simulink model "PMSM_HFI_PulseCos_Continuouse"  (R2022b)
settings: Solver=ode45  StartTime=0.0  StopTime=3  RelTol=1e-3  EnableMultiTasking=on
libraries: dsparch4 x6, spsVoltageMeasurementLib x3, spsUniversalBridgeLib x2, spsGroundLib x1, spsPermanentMagnetSynchronousMachineLib x1, simulink x1, spsThreePhaseVIMeasurementLib x1, spsDCVoltageSourceLib x1, spspowerguiLib x1
settings Model: Creator=lovejing  LastModifiedBy=yll
settings SolverCC: ZeroCrossAlgorithm=Adaptive  AlgebraicLoopSolver=TrustRegion
settings DataIOCC: LimitDataPoints=on  SaveFormat=Array  SignalLoggingSaveFormat=ModelDataLogs  ReturnWorkspaceOutputs=off
settings OptimizationCC: ExpressionDepthLimit=2147483647  LifeSpan=inf
settings DebuggingCC: UnderspecifiedInitializationDetection=Classic  MergeDetectMultiDrivingBlocksExec=none  SolverPrmCheckMsg=warning  FcnCallInpInsideContextMsg=warning  UnconnectedInputMsg=warning  UnconnectedOutputMsg=warning  UnconnectedLineMsg=warning  StateNameClashWarn=warning  SFUnexpectedBacktrackingDiag=warning  SFNoUnconditionalDefaultTransitionDiag=warning  SFExecutionAtInitializationDiag=none  SFMachineParentedDataDiag=warning  ArithmeticOperatorsInVariantConditions=warning
settings HardwareCC: ProdBitPerPointer=32  ProdBitPerSizeT=32  ProdBitPerPtrDiffT=32  ProdLargestAtomicFloat=None  ProdIntDivRoundTo=Undefined  ProdEndianess=Unspecified  ProdWordSize=32  ProdHWDeviceType=32-bit Generic
settings ModelReferenceCC: PropagateSignalLabelsOutOfModel=off
settings SFSimCC: SimUseLocalCustomCode=off  CustomCodeUndefinedFunction=UseInterfaceOnly
settings RTWCC: RTWUseLocalCustomCode=off
settings CodeAppCC: StateflowObjectComments=on
settings GRTTargetCC: TargetLangStandard=C89/C90 (ANSI)  CombineOutputUpdateFcns=off  GRTInterface=on
settings ConfigComp: CovMetricSettings=dw  CovSaveCumulativeToWorkspaceVar=on  CovSaveSingleToWorkspaceVar=on  CovExternalEMLEnable=off  CovSFcnEnable=off
settings SimscapeCC: SimscapeNormalizeSystem=off

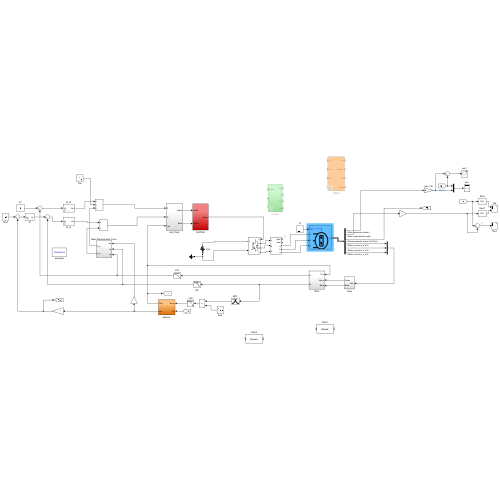
[thumbnail: Simulink's stored preview of the top-level diagram]
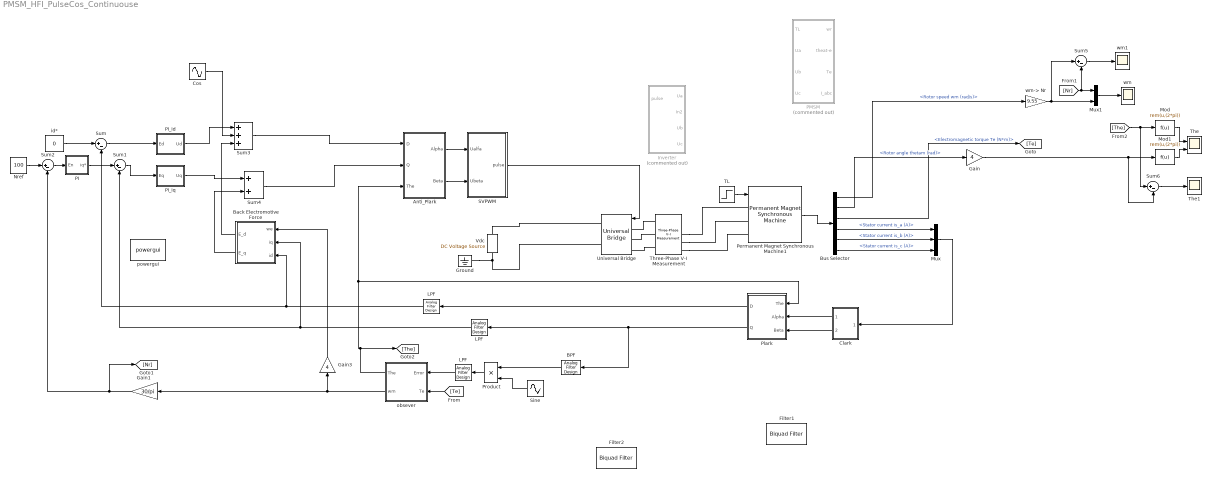
== system PMSM_HFI_PulseCos_Continuouse ==
  " LPF" : dsparch4/Analog Filter Design  method=Butterworth  filttype=Lowpass  N=1  Wlo=942  Whi=80  Rp=2  Rs=40
  Anti_Plark : Subsystem
  BPF : dsparch4/Analog Filter Design  method=Butterworth  filttype=Bandpass  N=2  Wlo=6200  Whi=6360  Rp=2  Rs=40
  Back Electromotive Force : Subsystem
  Bus Selector : BusSelector  OutputSignals=Rotor speed wm (rad/s),Rotor angle thetam (rad),Electromagnetic torque Te (N*m),Stator current is_a (A),Stator current is_b (A),Stator current is_c (A)
  Clark : Subsystem
  Cos : Sin  Amplitude=20  Frequency=6280  Phase=pi/2  SampleTime=0
  Filter1 : dsparch4/Biquad Filter  Tag=BlockMethodSubSystem  FilterSource=Dialog parameters  CoeffSource=Specify via dialog  FilterObject=BQF  IIRFiltStruct=Direct form II  BiQuadCoeffs=[1 0 -1 1 -1.99827576792918582 0.999875701454450927;1 0 -1 1 -1.99836499980206295 0.999879080975449419;1 0 -1 1 -1.99803610170332835 0.999633631467209849;1 0 -1 1 -1.99812710154029682 0.999643098504342187;1 0 -1 1 -1.99781763221036179 0.99941068343367212;1 0 -1 1 -1.99790443799382444 0.999424361176048381;1 0 -1 1 -1.99763159357438957 0.999218332257679753;1 0 -1 1 -1.99770783357569925 0.999233511136148667;1 0 -1 1 -1.99748738637941559 0.999066314462234151;1 0 -1 1 -1.99754699818338244 0.999079988713626688;1 0 -1 1 -1.9973920922120505 0.998962122228290506;1 0 -1 1 -1.99743006957830049 0.998971584387099765;1 0 -1 1 -1.99735014806338107 0.998910653324007525;1 0 -1 1 -1.99736319098991588 0.99891403010315738]  ScaleValues=[0.000547534400617177147;0.000547534400617177147;0.000547468966985179494;0.000547468966985179494;0.000547408518068997194;0.000547408518068997194;0.000547356078689129684;0.000547356078689129684;0.000547314270478672362;0.000547314270478672362;0.000547285181986175264;0.000547285181986175264;0.000547270265506675873;0.000547270265506675873;1]  IC=0  ICnum=0  ICden=0  a0Flag=Warning  optimizeScaleValues=on  ScaleValueMode=Specify via input port (g)  InputProcessing=Columns as channels (frame based)  roundingMode=Floor  overflowMode=off  scaleValueFracLength=14  denProdOutputFracLength=30  denAccumFracLength=30  secondMemoryFracLength=15
  Filter2 : dsparch4/Biquad Filter  Tag=BlockMethodSubSystem  FilterSource=Dialog parameters  CoeffSource=Specify via dialog  FilterObject=BQF  IIRFiltStruct=Direct form II  BiQuadCoeffs=[1 0 -1 1 -1.99827576792918582 0.999875701454450927;1 0 -1 1 -1.99836499980206295 0.999879080975449419;1 0 -1 1 -1.99803610170332835 0.999633631467209849;1 0 -1 1 -1.99812710154029682 0.999643098504342187;1 0 -1 1 -1.99781763221036179 0.99941068343367212;1 0 -1 1 -1.99790443799382444 0.999424361176048381;1 0 -1 1 -1.99763159357438957 0.999218332257679753;1 0 -1 1 -1.99770783357569925 0.999233511136148667;1 0 -1 1 -1.99748738637941559 0.999066314462234151;1 0 -1 1 -1.99754699818338244 0.999079988713626688;1 0 -1 1 -1.9973920922120505 0.998962122228290506;1 0 -1 1 -1.99743006957830049 0.998971584387099765;1 0 -1 1 -1.99735014806338107 0.998910653324007525;1 0 -1 1 -1.99736319098991588 0.99891403010315738]  ScaleValues=[0.000547534400617177147;0.000547534400617177147;0.000547468966985179494;0.000547468966985179494;0.000547408518068997194;0.000547408518068997194;0.000547356078689129684;0.000547356078689129684;0.000547314270478672362;0.000547314270478672362;0.000547285181986175264;0.000547285181986175264;0.000547270265506675873;0.000547270265506675873;1]  IC=0  ICnum=0  ICden=0  a0Flag=Warning  optimizeScaleValues=on  ScaleValueMode=Specify via input port (g)  InputProcessing=Columns as channels (frame based)  roundingMode=Floor  overflowMode=off  scaleValueFracLength=14  denProdOutputFracLength=30  denAccumFracLength=30  secondMemoryFracLength=15
  Gain : Gain  Gain=4
  Gain1 : Gain  Gain=30/pi
  Gain3 : Gain  Gain=4
  Ground : spsGroundLib/Ground  LConnTagsString=a
  Inverter : Subsystem  Commented=on
      settings: PortSchema="{\"entries\":[{\"content\":{\"sides\":[{\"content\":{\"connectorIds\":[\"In1\",\"LConn1\",\"LConn2\"]},\"type\":\"ConnectorPlacement.EquallySpacedRectSide\",\"uuid\":\"4e818927-345e-4f01-8e72-8098c662edc2\"},{\"content\":{\"connectorIds\":[\"Out1\",\"In2\",\"Out2\",\"Out3\"],\"side\":\"RIGHT\"},\"type\":\"ConnectorPlacement.EquallySpacedRectSide\",\"uuid\":\"f77f2109-fd93-4188-b06e-da3c9e8aa1ae\"},{\"content\":{\"connectorIds\":[],\"side\":\"TOP\"},\"type\":\"ConnectorPlacement.EquallySpacedRectSide\",\"uuid\":\"a2773a45-0f31-47fa-94c1-50539ffbc16b\"}]},\"type\":\"ConnectorPlacement.EquallySpacedConnector\",\"uuid\":\"32311cb9-9857-42c7-bd27-5d83894cf80f\"}],\"packageUris\":[\"http://schema.mathworks.com/mf0/Connector/R2020b\"],\"version\":\"1.0\"}"
  LPF : dsparch4/Analog Filter Design  method=Butterworth  filttype=Lowpass  N=1  Wlo=942  Whi=80  Rp=2  Rs=40
  "LPF " : dsparch4/Analog Filter Design  method=Butterworth  filttype=Lowpass  N=1  Wlo=942  Whi=80  Rp=2  Rs=40
  Mod : Fcn  Expr=rem(u,(2*pi))
  Mod1 : Fcn  Expr=rem(u,(2*pi))
  Mux : Mux  Inputs=3
  Mux1 : Mux  Inputs=2
  Nref : Constant  Value=100
  PI : Subsystem  mask{Knp=0.4, Kni=2}
  PI_id : Subsystem  mask{Kip=40, Kii=1}
  PI_iq : Subsystem  mask{Kip=40, Kii=1}
  PMSM : Subsystem  Commented=on  mask{Ld=0.0052, R=0.33, Lq=0.0174, kf=0.646, p=2, F=0, J=0.008}
  Permanent Magnet Synchronous Machine1 : spsPermanentMagnetSynchronousMachineLib/Permanent Magnet Synchronous Machine  NbPhases=3  FluxDistribution=Sinusoidal  RotorType=Salient-pole  MechanicalLoad=Torque Tm  PresetModel=No  ShowDetailedParameters=on  MeasurementBus=off  Resistance=0.02  Inductance=8.5e-3  dqInductances=[0.002 0.004]  La=Motor_Ld_Indctances  MachineConstant=Flux linkage established by magnets (V.s)  Flux=0.08  VoltageCst=58.0416  TorqueCst=0.48  Flat=120  Mechanical=[0.003 0 4 0]  PolePairs=4  InitialConditions=[0,0,0,0]  InitialConditions5ph=[0 0 0 0 0 0]  RefAngle=Aligned with phase A axis (original Park)  IterativeDiscreteModel=Trapezoidal robust  TsBlock=-1  TsPowergui=0
  Plark : Subsystem
  Product : Product
  SVPWM : Subsystem
  "Sine " : Sin  Frequency=6280  SampleTime=0
  Sum{,1..2,5..6} (5 alike) : Sum  Inputs=|+-
  Sum3 : Sum  Inputs=+++
  Sum4 : Sum
  TL : Step  Time=0.05  After=0  SampleTime=0
  The : Scope  NumInputPorts=2
  The1 : Scope
  Three-Phase V-I Measurement : spsThreePhaseVIMeasurementLib/Three-Phase V-I Measurement  VoltageMeasurement=phase-to-ground  SetLabelV=off  LabelV=Vabc  Vpu=off  VpuLL=off  CurrentMeasurement=yes  SetLabelI=off  LabelI=Iabc  Ipu=off  Pbase=100e6  Vbase=500e3  OutputType=Complex  PhasorSimulation=off  PSBequivalent=0
  Universal Bridge : spsUniversalBridgeLib/Universal Bridge  Arms=3  SnubberResistance=1e5  SnubberCapacitance=inf  Device=IGBT / Diodes  Ron=1e-3  Lon=0  ForwardVoltages="[  0  0  ]"  ForwardVoltage=0  GTOparameters=[ 10e-6 , 20e-6 ]  IGBTparameters=[ 1e-6 , 2e-6 ]  Measurements=None  Measurements_2=None  converterType=Rectifier
  "Vdc " : spsDCVoltageSourceLib/DC Voltage Source  Amplitude=311  Measurements=None
  id* : Constant  Value=0
  obsever : Subsystem
  powergui : spspowerguiLib/powergui  Priority=1  SimulationMode=Continuous  SampleTime=1e-6  frequency=60  Iterations=50  frequencyindice=0  Pbase=100e6  ErrMax=1e-4  UnitsV=kV  UnitsW=MW  buscounter=0  FunctionMessages=off  echomessages=off  EnableUseOfTLC=off  CurrentSourceSwitches=off  DisableSnubberDevices=off  DisableRonSwitches=off  DisableVfSwitches=off  DisplayEquations=off  AutomaticDiscreteSolvers=off  SolverType=Tustin/Backward Euler (TBE)  Interpol=off  ExternalGateDelay=off  methode=off  Ts=100  x0status=blocks  SPID=off  SwTol=0  HookPort=off  NonlinearTolerance=1e-4  nMaxIteration=100  ContinueOnMaxIteration=off  RestoreLinks=warning  ResistiveCurrentMeasurement=off  Frange=[0:2:500]  Ylog=off  Xlog=on  ShowGrid=off  save=off  variable=ZData  structure=0  ZoomFFT=off  StartTime=0.0  cycles=1  DisplayStyle=1  fundamental=60  FreqAxis=off  MaxFrequency=1000  frequencyindicesteady=1  RmsSteady=1  display=off
  wm : Scope
  wm-> Nr : Gain  Gain=9.55
  wm1 : Scope
  wires:
  Gain/1 -> Sum6/2, Mod1/1
  Bus Selector/3 -> [Te]  "<Electromagnetic torque Te (N*m)>"
  Bus Selector/4 -> Mux/1  "<Stator current is_a (A)>"
  TL/1 -> Permanent Magnet Synchronous Machine1/1
  BPF/1 -> Product/1
  SVPWM/1(pulse) -> Universal Bridge/1
  " LPF"/1 -> obsever/1(Error)
  [Te] -> obsever/2(Te)
  "Sine "/1 -> Product/2
  wm-> Nr/1 -> Sum5/1, Mux1/2
  [The] -> Sum6/1, Mod/1
  [Nr] -> Sum5/2, Mux1/1
  Plark/2(Q) -> BPF/1, "LPF "/1
  Gain1/1 -> [Nr], Sum2/2
  PI/1(iq*) -> Sum1/1
  "LPF "/1 -> Back Electromotive Force/2(iq), Sum1/2
  id*/1 -> Sum/1
  Plark/1(D) -> LPF/1
  Mod/1 -> The/1
  Sum3/1 -> Anti_Plark/1(D)
  Anti_Plark/1(Alpha) -> SVPWM/1(Ualfa)
  Clark/2(Beta) -> Plark/3(Beta)
  Mux1/1 -> wm/1
  Clark/1(Alpha) -> Plark/2(Alpha)
  Sum5/1 -> wm1/1
  PI_id/1(Ud) -> Sum3/1
  LPF/1 -> Back Electromotive Force/3(id), Sum/2
  Permanent Magnet Synchronous Machine1/1 -> Bus Selector/1
  Sum1/1 -> PI_iq/1(Eq)
  Sum/1 -> PI_id/1(Ed)
  Sum2/1 -> PI/1(En)
  Nref/1 -> Sum2/1
  Anti_Plark/2(Beta) -> SVPWM/2(Ubeta)
  Bus Selector/2 -> Gain/1  "<Rotor angle thetam (rad)>"
  Bus Selector/6 -> Mux/3  "<Stator current is_c (A)>"
  Bus Selector/5 -> Mux/2  "<Stator current is_b (A)>"
  Mod1/1 -> The/2
  obsever/1(The) -> [The], Plark/1(The), Anti_Plark/3(The)
  Product/1 -> " LPF"/1
  Mux/1 -> Clark/1(ABC)
  Sum6/1 -> The1/1
  Bus Selector/1 -> wm-> Nr/1  "<Rotor speed wm (rad/s)>"
  Cos/1 -> Sum3/2
  Sum4/1 -> Anti_Plark/2(Q)
  PI_iq/1(Uq) -> Sum4/1
  Back Electromotive Force/1(E_d) -> Sum3/3
  Back Electromotive Force/2(E_q) -> Sum4/2
  obsever/2(wm) -> Gain3/1, Gain1/1
  Gain3/1 -> Back Electromotive Force/1(we)
  connections:
  "Vdc "/LConn1 -- Universal Bridge/RConn2 -- Ground/LConn1
  Universal Bridge/RConn1 -- "Vdc "/RConn1
  Three-Phase V-I Measurement/LConn2 -- Universal Bridge/LConn2
  Three-Phase V-I Measurement/RConn1 -- Permanent Magnet Synchronous Machine1/LConn1
  Three-Phase V-I Measurement/RConn2 -- Permanent Magnet Synchronous Machine1/LConn2
  Three-Phase V-I Measurement/LConn3 -- Universal Bridge/LConn3
  Three-Phase V-I Measurement/RConn3 -- Permanent Magnet Synchronous Machine1/LConn3
  Three-Phase V-I Measurement/LConn1 -- Universal Bridge/LConn1

== system PMSM_HFI_PulseCos_Continuouse/Anti_Plark ==
  D : Inport
  Q : Inport  Port=2
  The : Inport  Port=3
  Mux : Mux  Inputs=3
  alpha : Fcn  Expr=u(1)*cos(u(3))-u(2)*sin(u(3))
  beta : Fcn  Expr=u(1)*sin(u(3))+u(2)*cos(u(3))
  Alpha : Outport
  Beta : Outport  Port=2
  wires:
  alpha/1 -> Alpha/1
  Q/1 -> Mux/2
  The/1 -> Mux/3
  D/1 -> Mux/1
  Mux/1 -> beta/1, alpha/1
  beta/1 -> Beta/1

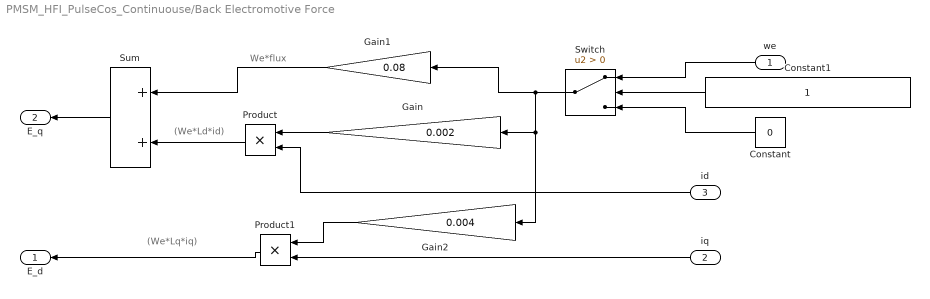
== system PMSM_HFI_PulseCos_Continuouse/Back Electromotive Force ==
  note: (We*Ld*id)
  note: We*flux
  note: (We*Lq*iq)
  we : Inport
  iq : Inport  Port=2
  id : Inport  Port=3
  Constant : Constant  Value=0
  Constant1 : Constant
  Gain : Gain  Gain=0.002
  Gain1 : Gain  Gain=0.08
  Gain2 : Gain  Gain=0.004
  Product : Product
  Product1 : Product
  Sum : Sum
  Switch : Switch  Criteria=u2 > Threshold  SaturateOnIntegerOverflow=off  InputSameDT=off
  E_d : Outport
  E_q : Outport  Port=2
  wires:
  Constant/1 -> Switch/3
  we/1 -> Switch/1
  Gain/1 -> Product/1
  Gain2/1 -> Product1/1
  iq/1 -> Product1/2
  id/1 -> Product/2
  Constant1/1 -> Switch/2
  Product/1 -> Sum/2
  Sum/1 -> E_q/1
  Gain1/1 -> Sum/1
  Product1/1 -> E_d/1
  Switch/1 -> Gain2/1, Gain/1, Gain1/1

== system PMSM_HFI_PulseCos_Continuouse/Clark ==
  ABC : Inport
  alpha : Fcn  Expr=(u(1)-0.5*(u(2)+u(3)))*2/3
  beta : Fcn  Expr=sqrt(3)/2*(u(2)-u(3))*2/3
  Alpha : Outport
  Beta : Outport  Port=2
  wires:
  alpha/1 -> Alpha/1
  ABC/1 -> beta/1, alpha/1
  beta/1 -> Beta/1

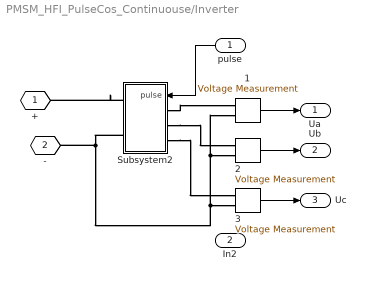
== system PMSM_HFI_PulseCos_Continuouse/Inverter ==
  pulse : Inport
  In2 : Inport  Port=2
  1 : spsVoltageMeasurementLib/Voltage Measurement  PhasorSimulation=off  OutputType=Complex  PSBequivalent=0
  2 : spsVoltageMeasurementLib/Voltage Measurement  PhasorSimulation=off  OutputType=Complex  PSBequivalent=0
  3 : spsVoltageMeasurementLib/Voltage Measurement  PhasorSimulation=off  OutputType=Complex  PSBequivalent=0
  Subsystem2 : Subsystem
  + : PMIOPort  Tag=PMCPort  Side=Left
  - : PMIOPort  Tag=PMCPort  Port=2  Side=Left
  Ua : Outport
  Ub : Outport  Port=2
  Uc : Outport  Port=3
  wires:
  3/1 -> Uc/1
  2/1 -> Ub/1
  1/1 -> Ua/1
  pulse/1 -> Subsystem2/1(pulse)
  connections:
  Subsystem2/LConn1 -- 1/LConn1
  -/RConn1 -- Subsystem2/RConn2 -- 3/LConn2 -- 2/LConn2 -- 1/LConn2
  Subsystem2/LConn2 -- 2/LConn1
  Subsystem2/LConn3 -- 3/LConn1
  Subsystem2/RConn1 -- +/RConn1

== system PMSM_HFI_PulseCos_Continuouse/PI ==
  En : Inport
  Gain : Gain  Gain=Kni
  Gain1 : Gain  Gain=Knp
  Integrator : Integrator
  Saturation : Saturate  UpperLimit=50  LowerLimit=-50
  Subtract : Sum
  iq* : Outport
  wires:
  En/1 -> Gain/1, Gain1/1
  Gain/1 -> Integrator/1
  Integrator/1 -> Subtract/1
  Gain1/1 -> Subtract/2
  Subtract/1 -> Saturation/1
  Saturation/1 -> iq*/1

== system PMSM_HFI_PulseCos_Continuouse/PI_id ==
  Ed : Inport
  Gain : Gain  Gain=Kii
  Gain1 : Gain  Gain=Kip
  Integrator : Integrator
  Saturation : Saturate  UpperLimit=10  LowerLimit=-10
  Subtract : Sum
  Ud : Outport
  wires:
  Ed/1 -> Gain/1, Gain1/1
  Gain/1 -> Integrator/1
  Integrator/1 -> Subtract/1
  Gain1/1 -> Subtract/2
  Subtract/1 -> Saturation/1
  Saturation/1 -> Ud/1

== system PMSM_HFI_PulseCos_Continuouse/PI_iq ==
  Eq : Inport
  Gain : Gain  Gain=Kii
  Gain1 : Gain  Gain=Kip
  Integrator : Integrator
  Saturation : Saturate  UpperLimit=100  LowerLimit=-100
  Subtract : Sum
  Uq : Outport
  wires:
  Eq/1 -> Gain/1, Gain1/1
  Gain/1 -> Integrator/1
  Integrator/1 -> Subtract/1
  Gain1/1 -> Subtract/2
  Subtract/1 -> Saturation/1
  Saturation/1 -> Uq/1

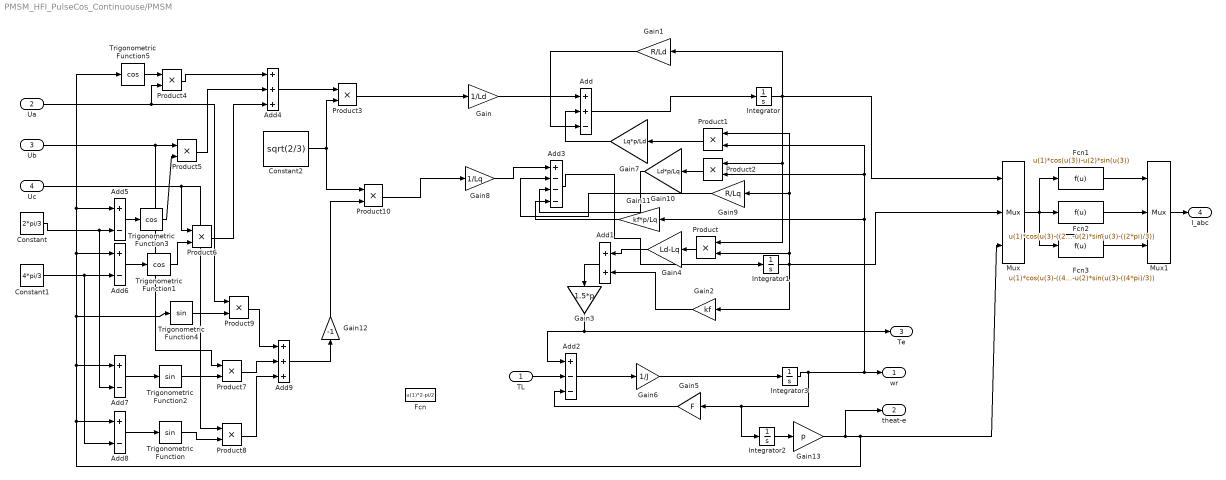
== system PMSM_HFI_PulseCos_Continuouse/PMSM ==
  TL : Inport
  Ua : Inport  Port=2
  Ub : Inport  Port=3
  Uc : Inport  Port=4
  Add : Sum  Inputs=++-
  Add1 : Sum
  Add2 : Sum  Inputs=+--
  Add3 : Sum  Inputs=+---
  Add4 : Sum  Inputs=+++
  Add{5..8} (4 alike) : Sum  Inputs=+-
  Add9 : Sum  Inputs=+++
  Constant : Constant  Value=2*pi/3
  Constant1 : Constant  Value=4*pi/3
  Constant2 : Constant  Value=sqrt(2/3)
  Fcn : Fcn  Expr=u(1)*2-pi/2
  Fcn1 : Fcn  Expr=u(1)*cos(u(3))-u(2)*sin(u(3))
  Fcn2 : Fcn  Expr=u(1)*cos(u(3)-((2*pi)/3))-u(2)*sin(u(3)-((2*pi)/3))
  Fcn3 : Fcn  Expr=u(1)*cos(u(3)-((4*pi)/3))-u(2)*sin(u(3)-((4*pi)/3))
  Gain : Gain  Gain=1/Ld
  Gain1 : Gain  Gain=R/Ld
  Gain10 : Gain  Gain=Ld*p/Lq
  Gain11 : Gain  Gain=kf*p/Lq
  Gain12 : Gain  Gain=-1
  Gain13 : Gain  Gain=p
  Gain2 : Gain  Gain=kf
  Gain3 : Gain  Gain=1.5*p
  Gain4 : Gain  Gain=Ld-Lq
  Gain5 : Gain  Gain=F
  Gain6 : Gain  Gain=1/J
  Gain7 : Gain  Gain=Lq*p/Ld
  Gain8 : Gain  Gain=1/Lq
  Gain9 : Gain  Gain=R/Lq
  Integrator{,1..3} (4 alike) : Integrator
  Mux : Mux  Inputs=3
  Mux1 : Mux  Inputs=3
  Product{,1..10} (11 alike) : Product  RndMeth=Zero
  Trigonometric Function : Trigonometry
  Trigonometric Function1 : Trigonometry  Operator=cos
  Trigonometric Function2 : Trigonometry
  Trigonometric Function3 : Trigonometry  Operator=cos
  Trigonometric Function4 : Trigonometry
  Trigonometric Function5 : Trigonometry  Operator=cos
  wr : Outport
  theat-e : Outport  Port=2
  Te : Outport  Port=3
  I_abc : Outport  Port=4
  wires:
  Add3/1 -> Integrator1/1
  Gain11/1 -> Add3/4
  Gain10/1 -> Add3/3
  Product2/1 -> Gain10/1
  Gain9/1 -> Add3/2
  Gain8/1 -> Add3/1
  Add/1 -> Integrator/1
  Gain7/1 -> Add/2
  Product1/1 -> Gain7/1
  Gain6/1 -> Integrator3/1
  Add2/1 -> Gain6/1
  Gain5/1 -> Add2/3
  TL/1 -> Add2/2
  Integrator3/1 -> wr/1, Product1/2, Product2/2, Gain11/1, Gain5/1, Integrator2/1
  Gain3/1 -> Add2/1, Te/1
  Add1/1 -> Gain3/1
  Gain2/1 -> Add1/2
  Gain4/1 -> Add1/1
  Product/1 -> Gain4/1
  Gain1/1 -> Add/3
  Integrator1/1 -> Product/2, Product1/1, Gain9/1, Gain2/1, Mux/2
  Integrator/1 -> Gain1/1, Product/1, Product2/1, Mux/1
  Gain/1 -> Add/1
  Constant2/1 -> Product3/2, Product10/1
  Add4/1 -> Product3/1
  Product3/1 -> Gain/1
  Constant/1 -> Add5/2, Add7/2
  Add5/1 -> Trigonometric Function3/1
  Constant1/1 -> Add6/2, Add8/2
  Add6/1 -> Trigonometric Function1/1
  Trigonometric Function5/1 -> Product4/1
  Ua/1 -> Product4/2, Product9/1
  Product4/1 -> Add4/1
  Ub/1 -> Product5/1, Product7/1
  Trigonometric Function3/1 -> Product5/2
  Product5/1 -> Add4/2
  Uc/1 -> Product6/1, Product8/1
  Trigonometric Function1/1 -> Product6/2
  Product6/1 -> Add4/3
  Add7/1 -> Trigonometric Function2/1
  Add8/1 -> Trigonometric Function/1
  Trigonometric Function2/1 -> Product7/2
  Trigonometric Function/1 -> Product8/2
  Trigonometric Function4/1 -> Product9/2
  Product9/1 -> Add9/1
  Product7/1 -> Add9/2
  Product8/1 -> Add9/3
  Add9/1 -> Gain12/1
  Gain12/1 -> Product10/2
  Product10/1 -> Gain8/1
  Gain13/1 -> Add8/1, Add7/1, Trigonometric Function5/1, Add5/1, Add6/1, Trigonometric Function4/1, Mux/3, theat-e/1
  Fcn3/1 -> Mux1/3
  Fcn2/1 -> Mux1/2
  Fcn1/1 -> Mux1/1
  Mux/1 -> Fcn2/1, Fcn1/1, Fcn3/1
  Mux1/1 -> I_abc/1
  Integrator2/1 -> Gain13/1

== system PMSM_HFI_PulseCos_Continuouse/Plark ==
  The : Inport
  Alpha : Inport  Port=2
  Beta : Inport  Port=3
  Mux : Mux  Inputs=3
  d : Fcn  Expr=u(1)*cos(u(3))+u(2)*sin(u(3))
  q : Fcn  Expr=-u(1)*sin(u(3))+u(2)*cos(u(3))
  D : Outport
  Q : Outport  Port=2
  wires:
  d/1 -> D/1
  Beta/1 -> Mux/2
  The/1 -> Mux/3
  Alpha/1 -> Mux/1
  Mux/1 -> q/1, d/1
  q/1 -> Q/1

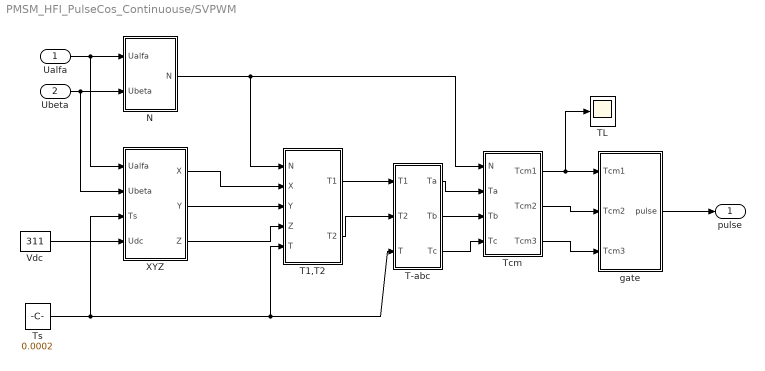
== system PMSM_HFI_PulseCos_Continuouse/SVPWM ==
  Ualfa : Inport
  Ubeta : Inport  Port=2
  N : Subsystem
  T-abc : Subsystem
  T1,T2 : Subsystem
  TL : Scope
  Tcm : Subsystem
  Ts : Constant  Value=0.0002  SampleTime=-1
  Vdc : Constant  Value=311
  XYZ : Subsystem
  gate : Subsystem
  pulse : Outport
  wires:
  Tcm/1(Tcm1) -> gate/1(Tcm1), TL/1
  T-abc/2(Tb) -> Tcm/3(Tb)
  T-abc/1(Ta) -> Tcm/2(Ta)
  T-abc/3(Tc) -> Tcm/4(Tc)
  T1,T2/1(T1) -> T-abc/1(T1)
  T1,T2/2(T2) -> T-abc/2(T2)
  XYZ/2(Y) -> T1,T2/3(Y)
  XYZ/1(X) -> T1,T2/2(X)
  XYZ/3(Z) -> T1,T2/4(Z)
  N/1(N) -> T1,T2/1(N), Tcm/1(N)
  Ts/1 -> T1,T2/5(T), T-abc/3(T), XYZ/3(Ts)
  gate/1(pulse) -> pulse/1
  Ualfa/1 -> N/1(Ualfa), XYZ/1(Ualfa)
  Ubeta/1 -> N/2(Ubeta), XYZ/2(Ubeta)
  Vdc/1 -> XYZ/4(Udc)
  Tcm/2(Tcm2) -> gate/2(Tcm2)
  Tcm/3(Tcm3) -> gate/3(Tcm3)

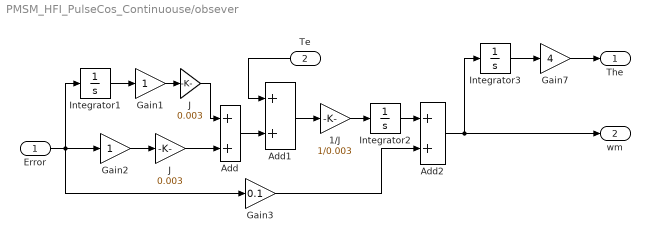
== system PMSM_HFI_PulseCos_Continuouse/obsever ==
  Error : Inport
  Te : Inport  Port=2
  1/J : Gain  Gain=1/0.003
  Add : Sum
  Add1 : Sum
  Add2 : Sum
  Gain1 : Gain
  Gain2 : Gain
  Gain3 : Gain  Gain=0.1
  Gain7 : Gain  Gain=4
  Integrator1 : Integrator
  Integrator2 : Integrator
  Integrator3 : Integrator
  J : Gain  Gain=0.003
  "J " : Gain  Gain=0.003
  The : Outport
  wm : Outport  Port=2
  wires:
  Error/1 -> Integrator1/1, Gain2/1, Gain3/1
  Integrator1/1 -> Gain1/1
  Add/1 -> Add1/2
  1/J/1 -> Integrator2/1
  Integrator2/1 -> Add2/1
  Add2/1 -> Integrator3/1, wm/1
  Gain2/1 -> "J "/1
  Gain1/1 -> J/1
  Gain3/1 -> Add2/2
  Integrator3/1 -> Gain7/1
  Add1/1 -> 1/J/1
  Te/1 -> Add1/1
  Gain7/1 -> The/1
  J/1 -> Add/1
  "J "/1 -> Add/2

== system PMSM_HFI_PulseCos_Continuouse/Inverter/Subsystem2 ==
  pulse : Inport
  Universal Bridge : spsUniversalBridgeLib/Universal Bridge  Arms=3  SnubberResistance=1e5  SnubberCapacitance=inf  Device=IGBT / Diodes  Ron=1e-3  Lon=0  ForwardVoltages="[  0  0  ]"  ForwardVoltage=0  GTOparameters=[ 10e-6 , 20e-6 ]  IGBTparameters=[ 1e-6 , 2e-6 ]  Measurements=None  Measurements_2=None  converterType=Rectifier
  Ua : PMIOPort  Tag=PMCPort  Side=Left
  Ub : PMIOPort  Tag=PMCPort  Port=2  Side=Left
  Uc : PMIOPort  Tag=PMCPort  Port=3  Side=Left
  + : PMIOPort  Tag=PMCPort  Port=4  Side=Right
  - : PMIOPort  Tag=PMCPort  Port=5  Side=Right
  wires:
  pulse/1 -> Universal Bridge/1
  connections:
  Universal Bridge/LConn1 -- Ua/RConn1
  Universal Bridge/LConn2 -- Ub/RConn1
  Universal Bridge/LConn3 -- Uc/RConn1
  +/RConn1 -- Universal Bridge/RConn1
  -/RConn1 -- Universal Bridge/RConn2

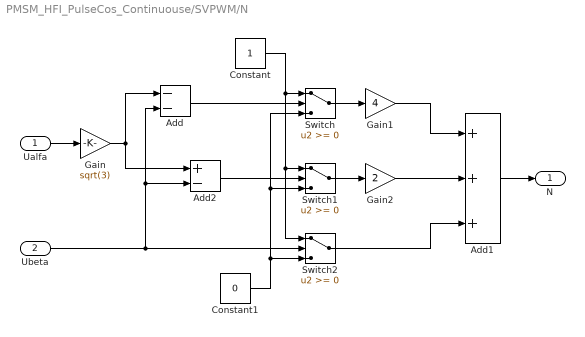
== system PMSM_HFI_PulseCos_Continuouse/SVPWM/N ==
  Ualfa : Inport
  Ubeta : Inport  Port=2
  Add : Sum  Inputs=--
  Add1 : Sum  Inputs=+++
  Add2 : Sum  Inputs=+-
  Constant : Constant
  Constant1 : Constant  Value=0
  Gain : Gain  Gain=sqrt(3)
  Gain1 : Gain  Gain=4
  Gain2 : Gain  Gain=2
  Switch : Switch  SaturateOnIntegerOverflow=off  InputSameDT=off
  Switch1 : Switch  SaturateOnIntegerOverflow=off  InputSameDT=off
  Switch2 : Switch  SaturateOnIntegerOverflow=off  InputSameDT=off
  N : Outport
  wires:
  Ualfa/1 -> Gain/1
  Add1/1 -> N/1
  Switch/1 -> Gain1/1
  Add/1 -> Switch/2
  Gain/1 -> Add/1, Add2/1
  Ubeta/1 -> Switch2/2, Add/2, Add2/2
  Gain1/1 -> Add1/1
  Switch2/1 -> Add1/3
  Add2/1 -> Switch1/2
  Switch1/1 -> Gain2/1
  Gain2/1 -> Add1/2
  Constant/1 -> Switch2/1, Switch1/1, Switch/1
  Constant1/1 -> Switch/3, Switch1/3, Switch2/3

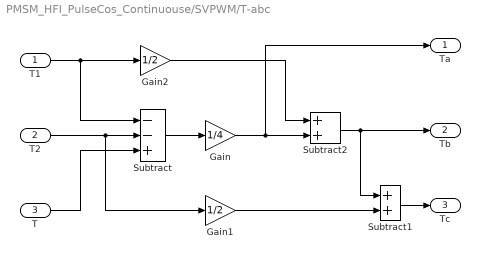
== system PMSM_HFI_PulseCos_Continuouse/SVPWM/T-abc ==
  T1 : Inport
  T2 : Inport  Port=2
  T : Inport  Port=3
  Gain : Gain  Gain=1/4
  Gain1 : Gain  Gain=1/2
  Gain2 : Gain  Gain=1/2
  Subtract : Sum  Inputs=--+
  Subtract1 : Sum
  Subtract2 : Sum
  Ta : Outport
  Tb : Outport  Port=2
  Tc : Outport  Port=3
  wires:
  T2/1 -> Subtract/2, Gain1/1
  T1/1 -> Subtract/1, Gain2/1
  T/1 -> Subtract/3
  Subtract/1 -> Gain/1
  Gain/1 -> Ta/1, Subtract2/2
  Gain2/1 -> Subtract2/1
  Subtract2/1 -> Tb/1, Subtract1/1
  Subtract1/1 -> Tc/1
  Gain1/1 -> Subtract1/2

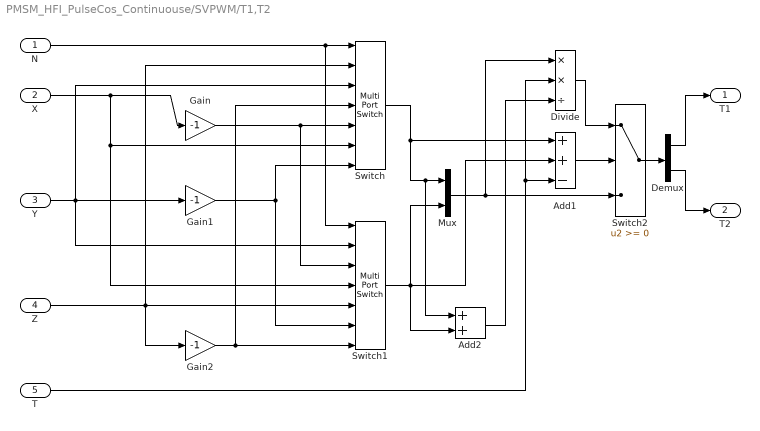
== system PMSM_HFI_PulseCos_Continuouse/SVPWM/T1,T2 ==
  N : Inport
  X : Inport  Port=2
  Y : Inport  Port=3
  Z : Inport  Port=4
  T : Inport  Port=5
  Add1 : Sum  Inputs=++-
  Add2 : Sum
  Demux : Demux  Outputs=2
  Divide : Product  Inputs=**/
  Gain : Gain  Gain=-1
  Gain1 : Gain  Gain=-1
  Gain2 : Gain  Gain=-1
  Mux : Mux  Inputs=2
  Switch : MultiPortSwitch  Inputs=6  SaturateOnIntegerOverflow=off  InputSameDT=off
  Switch1 : MultiPortSwitch  Inputs=6  SaturateOnIntegerOverflow=off  InputSameDT=off
  Switch2 : Switch  SaturateOnIntegerOverflow=off  InputSameDT=off
  T1 : Outport
  T2 : Outport  Port=2
  wires:
  Y/1 -> Switch/3, Gain1/1, Switch1/2
  Z/1 -> Switch/2, Switch1/5, Gain2/1
  X/1 -> Gain/1, Switch1/4, Switch/6
  Gain/1 -> Switch/5, Switch1/3
  Gain2/1 -> Switch/4, Switch1/7
  Gain1/1 -> Switch1/6, Switch/7
  Switch/1 -> Add1/1, Mux/1, Add2/1
  Switch1/1 -> Mux/2, Add1/2, Add2/2
  Mux/1 -> Divide/1, Switch2/3
  Switch2/1 -> Demux/1
  Demux/1 -> T1/1
  Demux/2 -> T2/1
  Add1/1 -> Switch2/2
  T/1 -> Add1/3, Divide/2
  Divide/1 -> Switch2/1
  Add2/1 -> Divide/3
  N/1 -> Switch/1, Switch1/1

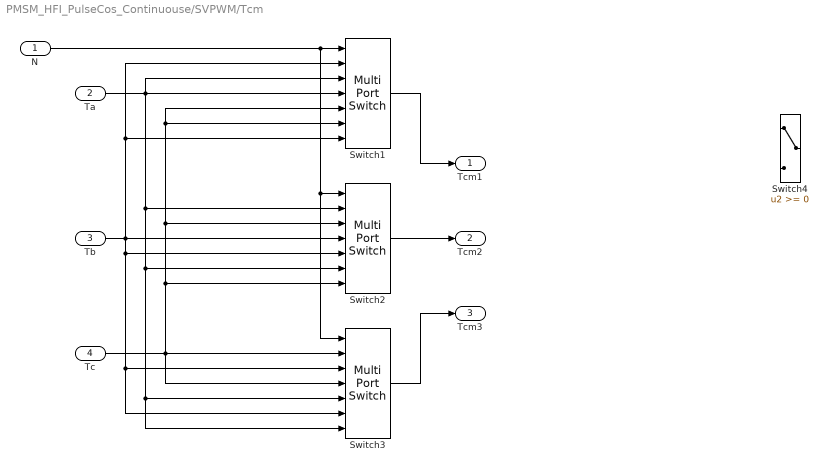
== system PMSM_HFI_PulseCos_Continuouse/SVPWM/Tcm ==
  N : Inport
  Ta : Inport  Port=2
  Tb : Inport  Port=3
  Tc : Inport  Port=4
  Switch1 : MultiPortSwitch  Inputs=6  SaturateOnIntegerOverflow=off  InputSameDT=off
  Switch2 : MultiPortSwitch  Inputs=6  SaturateOnIntegerOverflow=off  InputSameDT=off
  Switch3 : MultiPortSwitch  Inputs=6  SaturateOnIntegerOverflow=off  InputSameDT=off
  Switch4 : Switch  SaturateOnIntegerOverflow=off  InputSameDT=off
  Tcm1 : Outport
  Tcm2 : Outport  Port=2
  Tcm3 : Outport  Port=3
  wires:
  Switch2/1 -> Tcm2/1
  Switch3/1 -> Tcm3/1
  Switch1/1 -> Tcm1/1
  Tb/1 -> Switch2/4, Switch2/5, Switch3/3, Switch3/6, Switch1/2, Switch1/7
  Tc/1 -> Switch3/2, Switch3/4, Switch2/3, Switch1/5, Switch1/6, Switch2/7
  Ta/1 -> Switch1/4, Switch1/3, Switch2/2, Switch2/6, Switch3/5, Switch3/7
  N/1 -> Switch1/1, Switch2/1, Switch3/1

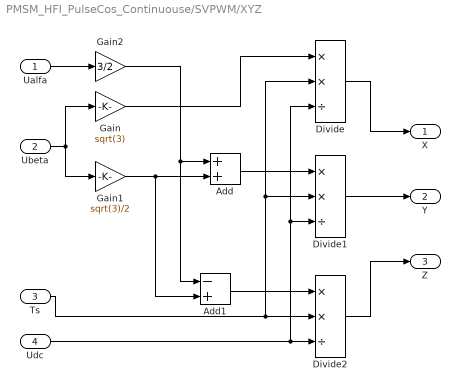
== system PMSM_HFI_PulseCos_Continuouse/SVPWM/XYZ ==
  Ualfa : Inport
  Ubeta : Inport  Port=2
  Ts : Inport  Port=3
  Udc : Inport  Port=4
  Add : Sum
  Add1 : Sum  Inputs=-+
  Divide : Product  Inputs=**/
  Divide1 : Product  Inputs=**/
  Divide2 : Product  Inputs=**/
  Gain : Gain  Gain=sqrt(3)
  Gain1 : Gain  Gain=sqrt(3)/2
  Gain2 : Gain  Gain=3/2
  X : Outport
  Y : Outport  Port=2
  Z : Outport  Port=3
  wires:
  Divide1/1 -> Y/1
  Divide/1 -> X/1
  Divide2/1 -> Z/1
  Ts/1 -> Divide2/2, Divide1/2, Divide/2
  Udc/1 -> Divide2/3, Divide1/3, Divide/3
  Ubeta/1 -> Gain/1, Gain1/1
  Ualfa/1 -> Gain2/1
  Gain/1 -> Divide/1
  Add/1 -> Divide1/1
  Gain1/1 -> Add/2, Add1/2
  Gain2/1 -> Add1/1, Add/1
  Add1/1 -> Divide2/1

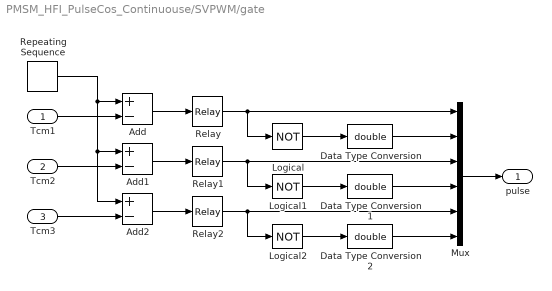
== system PMSM_HFI_PulseCos_Continuouse/SVPWM/gate ==
  Tcm1 : Inport
  Tcm2 : Inport  Port=2
  Tcm3 : Inport  Port=3
  Add : Sum  Inputs=+-
  Add1 : Sum  Inputs=+-
  Add2 : Sum  Inputs=+-
  Data Type Conversion : DataTypeConversion  OutDataTypeStr=double  SaturateOnIntegerOverflow=off  RndMeth=Floor
  Data Type Conversion1 : DataTypeConversion  OutDataTypeStr=double  SaturateOnIntegerOverflow=off  RndMeth=Floor
  Data Type Conversion2 : DataTypeConversion  OutDataTypeStr=double  SaturateOnIntegerOverflow=off  RndMeth=Floor
  Logical : Logic  Operator=NOT  AllPortsSameDT=off  OutDataTypeStr=boolean
  Logical1 : Logic  Operator=NOT  AllPortsSameDT=off  OutDataTypeStr=boolean
  Logical2 : Logic  Operator=NOT  AllPortsSameDT=off  OutDataTypeStr=boolean
  Mux : Mux  Inputs=6
  Relay : Relay
  Relay1 : Relay
  Relay2 : Relay
  Repeating Sequence : simulink/Sources/Repeating Sequence  rep_seq_t=[0 0.00005 0.0001]  rep_seq_y=[0 0.0001 0]
  pulse : Outport
  wires:
  Tcm1/1 -> Add/2
  Tcm2/1 -> Add1/2
  Tcm3/1 -> Add2/2
  Repeating Sequence/1 -> Add2/1, Add1/1, Add/1
  Add2/1 -> Relay2/1
  Add1/1 -> Relay1/1
  Add/1 -> Relay/1
  Relay/1 -> Mux/1, Logical/1
  Relay1/1 -> Mux/3, Logical1/1
  Relay2/1 -> Mux/5, Logical2/1
  Data Type Conversion/1 -> Mux/2
  Logical/1 -> Data Type Conversion/1
  Data Type Conversion1/1 -> Mux/4
  Logical1/1 -> Data Type Conversion1/1
  Data Type Conversion2/1 -> Mux/6
  Logical2/1 -> Data Type Conversion2/1
  Mux/1 -> pulse/1
